simulink model "BirdModel"  (R2023b)
settings: Solver=VariableStepAuto  StartTime=0.0  StopTime=100.0  RelTol=1e-3
values from neighbouring files (symbols this model uses):
  I = 2119    [Bird.m]    (also in BirdNoSim.m; DelaySweep.mat; NoiseSweep.mat; bird__pd_control.m = 0.002119)
  Ki = K    (= 9)    [Bird.m]
  Kp = K*tauC    (= 360)    [Bird.m]
  tauP = 69.7    [Bird.m]    (also in BirdNoSim.m = 0.0697)
settings Model: Creator=haydenwalker  LastModifiedBy=haydenwalker

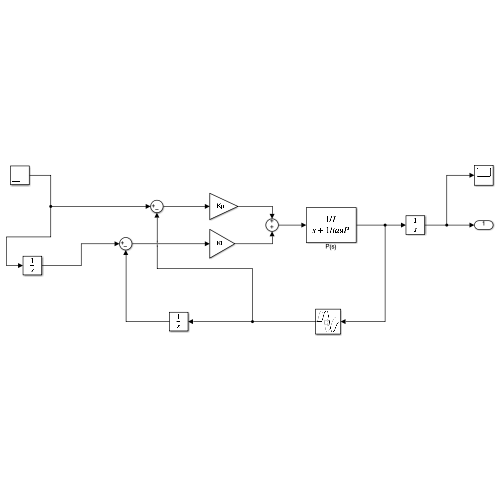
[thumbnail: Simulink's stored preview of the top-level diagram]
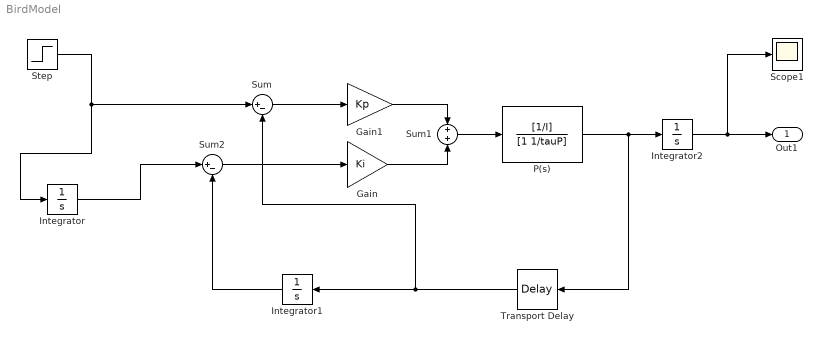
== system BirdModel ==
  Gain : Gain  Gain=Ki
  Gain1 : Gain  Gain=Kp
  Integrator : Integrator
  Integrator1 : Integrator
  Integrator2 : Integrator
  P(s) : TransferFcn  Numerator=[1/I]  Denominator=[1 1/tauP]
  Scope1 : Scope
  Step : Step  SampleTime=0
  Sum : Sum  Inputs=|+-
  Sum1 : Sum  Inputs=+|+
  Sum2 : Sum  Inputs=|+-
  Transport Delay : TransportDelay  DelayTime=0
  Out1 : Outport
  wires:
  Gain1/1 -> Sum1/1
  Gain/1 -> Sum1/2
  Sum1/1 -> P(s)/1
  P(s)/1 -> Transport Delay/1, Integrator2/1
  Step/1 -> Sum/1, Integrator/1
  Integrator/1 -> Sum2/1
  Integrator1/1 -> Sum2/2
  Sum2/1 -> Gain/1
  Sum/1 -> Gain1/1
  Transport Delay/1 -> Integrator1/1, Sum/2
  Integrator2/1 -> Scope1/1, Out1/1
